simulink model "AntiWindUp_model"  (R2022b)
settings: Solver=VariableStepAuto  StartTime=0.0  StopTime=100  RelTol=1e-3
values from neighbouring files (symbols this model uses):
  Kd = 1.6797    [AntiWindUp.m]
  Ki = 0.5372    [AntiWindUp.m]
  Kp = 1.4968    [AntiWindUp.m]
settings Model: Creator=Akash  LastModifiedBy=Akash

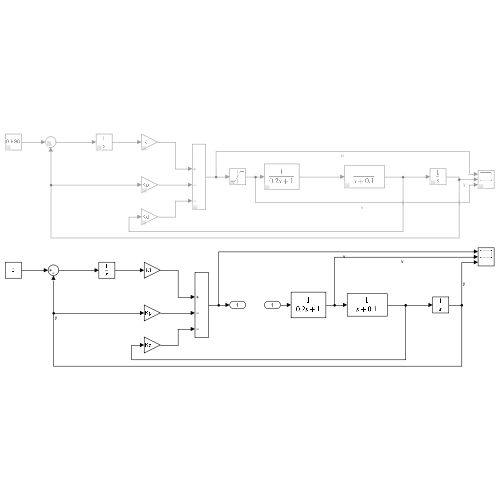
[thumbnail: Simulink's stored preview of the top-level diagram]
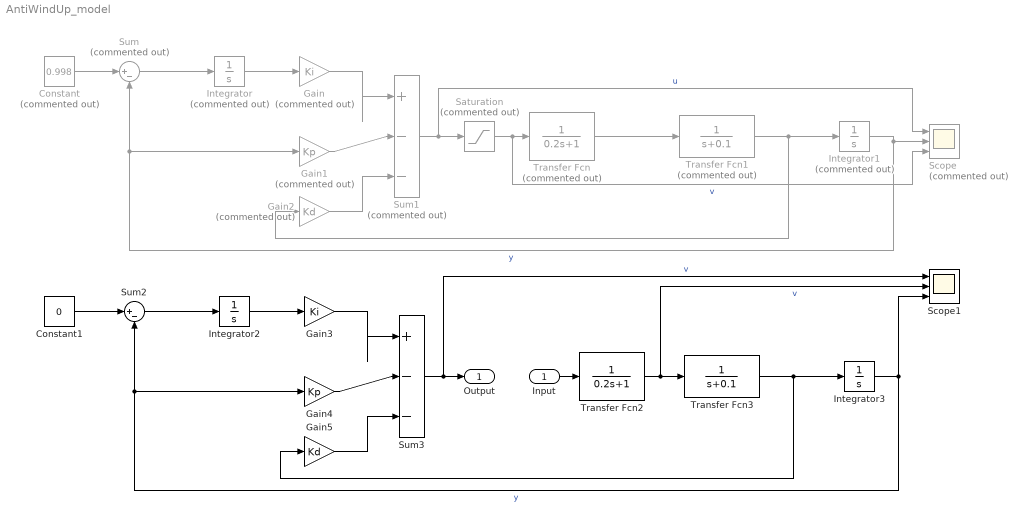
== system AntiWindUp_model ==
  Input : Inport
  Constant : Constant  Commented=on  Value=0.998
  Constant1 : Constant  Value=0
  Gain : Gain  Commented=on  Gain=Ki
  Gain1 : Gain  Commented=on  Gain=Kp
  Gain2 : Gain  Commented=on  Gain=Kd
  Gain3 : Gain  Gain=Ki
  Gain4 : Gain  Gain=Kp
  Gain5 : Gain  Gain=Kd
  Integrator : Integrator  Commented=on
  Integrator1 : Integrator  Commented=on
  Integrator2 : Integrator
  Integrator3 : Integrator
  Saturation : Saturate  Commented=on  UpperLimit=0.1  LowerLimit=-0.1
  Scope : Scope  Commented=on  NumInputPorts=3
  Scope1 : Scope  NumInputPorts=3
  Sum : Sum  Commented=on  Inputs=|+-
  Sum1 : Sum  Commented=on  Inputs=|+--
  Sum2 : Sum  Inputs=|+-
  Sum3 : Sum  Inputs=|+--
  Transfer Fcn : TransferFcn  Commented=on  Numerator=1  Denominator=[0.2 1]
  Transfer Fcn1 : TransferFcn  Commented=on  Numerator=1  Denominator=[1 0.1]
  Transfer Fcn2 : TransferFcn  Numerator=1  Denominator=[0.2 1]
  Transfer Fcn3 : TransferFcn  Numerator=1  Denominator=[1 0.1]
  Output : Outport
  wires:
  Sum/1 -> Integrator/1
  Integrator/1 -> Gain/1
  Transfer Fcn/1 -> Transfer Fcn1/1
  Transfer Fcn1/1 -> Gain2/1, Integrator1/1
  Gain/1 -> Sum1/1
  Gain1/1 -> Sum1/2
  Gain2/1 -> Sum1/3
  Integrator1/1 -> Gain1/1, Sum/2, Scope/2  "y"
  Sum1/1 -> Scope/1, Saturation/1  "u"
  Saturation/1 -> Scope/3, Transfer Fcn/1  "v"
  Constant/1 -> Sum/1
  Transfer Fcn2/1 -> Scope1/2, Transfer Fcn3/1  "v"
  Sum2/1 -> Integrator2/1
  Gain5/1 -> Sum3/3
  Integrator3/1 -> Scope1/3, Gain4/1, Sum2/2  "y"
  Transfer Fcn3/1 -> Gain5/1, Integrator3/1
  Sum3/1 -> Scope1/1, Output/1  "v"
  Integrator2/1 -> Gain3/1
  Gain4/1 -> Sum3/2
  Gain3/1 -> Sum3/1
  Input/1 -> Transfer Fcn2/1
  Constant1/1 -> Sum2/1
